simulink model "ThreePhaseInverter"  (R2019b)
settings: Solver=VariableStepAuto  StartTime=0.0  StopTime=1/50*20  RelTol=1e-9
undefined symbols (not defined in the file or in its folder): out
libraries: simulink x4, cstblocks x3
settings Model: Creator=reichyga  LastModifiedBy=reichyga
settings HardwareCC: ProdBitPerLong=64  ProdHWDeviceType=Intel->x86-64 (Linux 64)

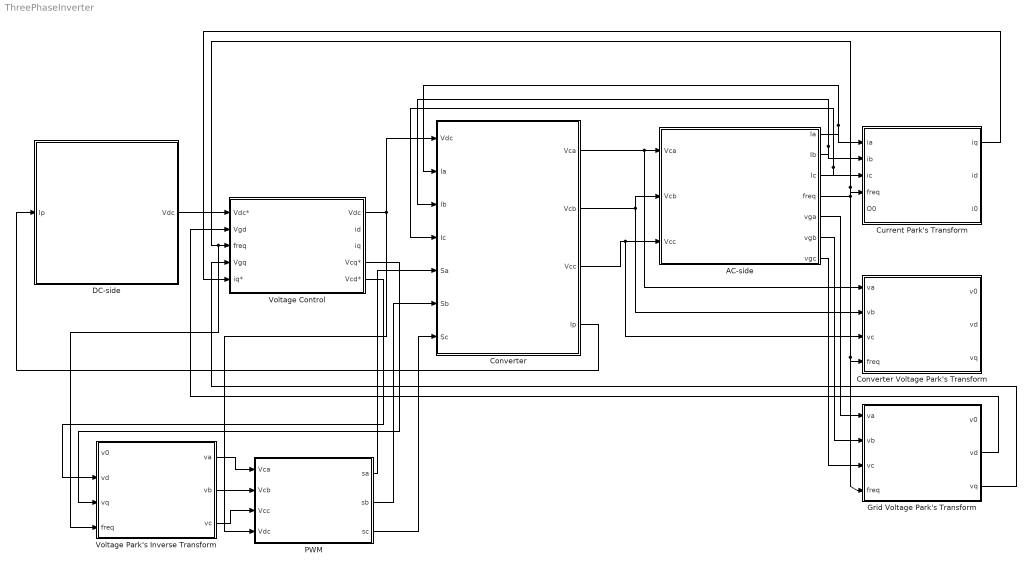
== system ThreePhaseInverter ==
  "AC-side " : Subsystem
  Converter : Subsystem
  Converter Voltage Park's Transform : Subsystem
  Current Park's Transform : Subsystem
  DC-side : Subsystem
  Grid Voltage Park's Transform : Subsystem
  PWM : Subsystem
  Voltage Control : Subsystem
  Voltage Park's Inverse Transform : Subsystem
  wires:
  "AC-side "/1(Ia) -> Converter/2(Ia), Current Park's Transform/1(ia)
  "AC-side "/3(Ic) -> Converter/4(Ic), Current Park's Transform/3(ic)
  Converter/1(Vca) -> Converter Voltage Park's Transform/1(va), "AC-side "/1("Vca ")
  Converter/2(Vcb) -> Converter Voltage Park's Transform/2(vb), "AC-side "/2(Vcb)
  Converter/3(Vcc) -> Converter Voltage Park's Transform/3(vc), "AC-side "/3(Vcc)
  Converter/4(Ip) -> DC-side/1(Ip)
  DC-side/1(Vdc) -> Voltage Control/1(Vdc*)
  "AC-side "/4(freq) -> Voltage Park's Inverse Transform/4("freq "), Voltage Control/3(freq), Current Park's Transform/4("freq "), Grid Voltage Park's Transform/4("freq "), Converter Voltage Park's Transform/4("freq ")
  "AC-side "/2(Ib) -> Converter/3(Ib), Current Park's Transform/2(ib)
  "AC-side "/5("vga ") -> Grid Voltage Park's Transform/1(va)
  "AC-side "/6(vgb) -> Grid Voltage Park's Transform/2(vb)
  "AC-side "/7("vgc ") -> Grid Voltage Park's Transform/3(vc)
  Grid Voltage Park's Transform/3(vq) -> Voltage Control/4(Vgq)
  Current Park's Transform/1("iq ") -> Voltage Control/5(iq*)
  Voltage Control/1(Vdc) -> PWM/4(Vdc), Converter/1(Vdc)
  Voltage Control/5(Vcd*) -> Voltage Park's Inverse Transform/2(vd)
  Voltage Control/4(Vcq*) -> Voltage Park's Inverse Transform/3(vq)
  Voltage Park's Inverse Transform/1("va ") -> PWM/1(Vca)
  Voltage Park's Inverse Transform/2(vb) -> PWM/2(Vcb)
  Voltage Park's Inverse Transform/3(vc) -> PWM/3(Vcc)
  PWM/1("sa ") -> Converter/5(Sa)
  PWM/2(sb) -> Converter/6(Sb)
  PWM/3(sc) -> Converter/7(Sc)
  Grid Voltage Park's Transform/2(vd) -> Voltage Control/2(Vgd)

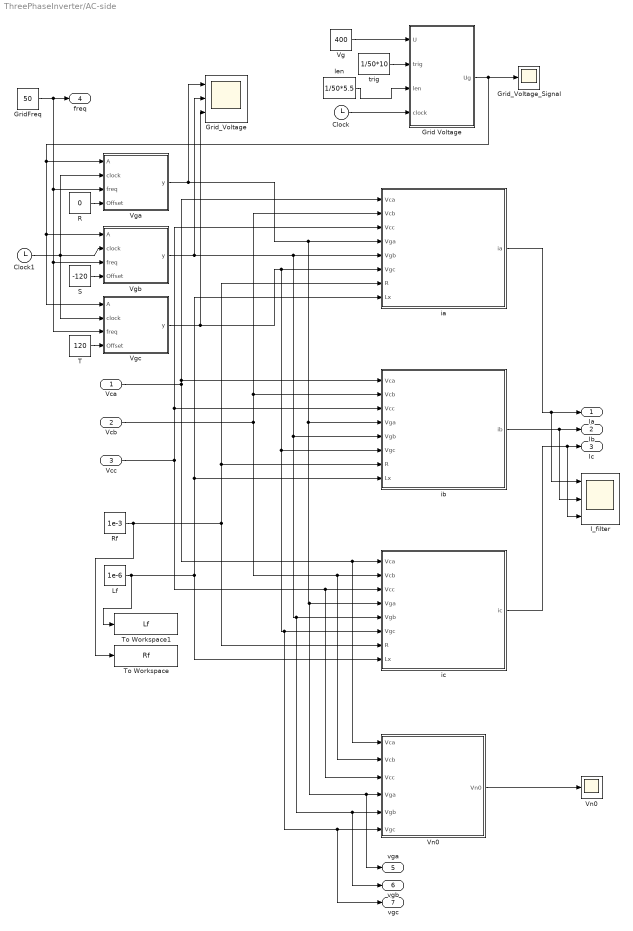
== system ThreePhaseInverter/AC-side  ==
  "Vca " : Inport
  Vcb : Inport  Port=2
  Vcc : Inport  Port=3
  Clock : Clock
  Clock1 : Clock
  Grid Voltage : MATLAB Function  TreatAsAtomicUnit=on
  "GridFreq " : Constant  Value=50
  Grid_Voltage : Scope  NumInputPorts=3
  "Grid_Voltage_Signal " : Scope
  I_filter : Scope  NumInputPorts=3
  "Lf " : Constant  Value=1e-6
  R : Constant  Value=0
  "Rf " : Constant  Value=1e-3
  S : Constant  Value=-120
  T : Constant  Value=120
  To Workspace : ToWorkspace  VariableName=Rf  SaveFormat=Timeseries  SampleTime=-1
  To Workspace1 : ToWorkspace  VariableName=Lf  SaveFormat=Timeseries  SampleTime=-1
  Vg : Constant  Value=400
  Vga : MATLAB Function  TreatAsAtomicUnit=on
  "Vgb " : MATLAB Function  TreatAsAtomicUnit=on
  Vgc : MATLAB Function  TreatAsAtomicUnit=on
  Vn0 : Subsystem
  "Vn0 " : Scope
  ia : Subsystem
  ib : Subsystem
  ic : Subsystem
  len : Constant  Value=1/50*5.5
  "trig " : Constant  Value=1/50*10
  Ia : Outport
  Ib : Outport  Port=2
  Ic : Outport  Port=3
  freq : Outport  Port=4
  "vga " : Outport  Port=5
  vgb : Outport  Port=6
  "vgc " : Outport  Port=7
  wires:
  Vn0/1("Vn0 ") -> "Vn0 "/1
  R/1 -> Vga/4(Offset)
  "Lf "/1 -> To Workspace1/1, ic/8(Lx), ib/8(Lx), ia/8(Lx)
  "Vca "/1 -> ib/1("Vca "), ia/1("Vca "), Vn0/1("Vca "), ic/1("Vca ")
  "Rf "/1 -> To Workspace/1, ib/7(R), ia/7(R), ic/7(R)
  Clock1/1 -> Vgc/2(clock), "Vgb "/2(clock), Vga/2(clock)
  Vcb/1 -> ib/2(Vcb), ia/2(Vcb), Vn0/2(Vcb), ic/2(Vcb)
  ic/1(ic) -> I_filter/3, Ic/1
  T/1 -> Vgc/4(Offset)
  ib/1(ib) -> I_filter/2, Ib/1
  Vg/1 -> Grid Voltage/1(U)
  Grid Voltage/1(Ug) -> Vgc/1(A), "Vgb "/1(A), Vga/1(A), "Grid_Voltage_Signal "/1
  Clock/1 -> Grid Voltage/4(clock)
  Vga/1(y) -> Grid_Voltage/1, "vga "/1, Vn0/4(Vga), ic/4(Vga), ib/4(Vga), ia/4(Vga)
  "Vgb "/1(y) -> Grid_Voltage/2, vgb/1, Vn0/5(Vgb), ic/5(Vgb), ib/5(Vgb), ia/5(Vgb)
  "trig "/1 -> Grid Voltage/2(trig)
  Vcc/1 -> Vn0/3(Vcc), ic/3(Vcc), ib/3(Vcc), ia/3(Vcc)
  "GridFreq "/1 -> Vga/3(freq), "Vgb "/3(freq), Vgc/3(freq), freq/1
  len/1 -> Grid Voltage/3(len)
  Vgc/1(y) -> Grid_Voltage/3, "vgc "/1, Vn0/6(Vgc), ic/6(Vgc), ib/6(Vgc), ia/6(Vgc)
  S/1 -> "Vgb "/4(Offset)
  ia/1(ia) -> I_filter/1, Ia/1

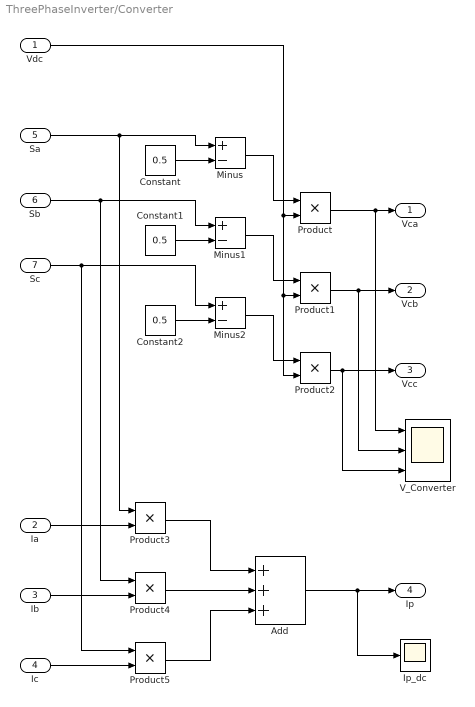
== system ThreePhaseInverter/Converter ==
  Vdc : Inport
  Ia : Inport  Port=2
  Ib : Inport  Port=3
  Ic : Inport  Port=4
  Sa : Inport  Port=5
  Sb : Inport  Port=6
  Sc : Inport  Port=7
  Add : Sum  Inputs=3
  Constant : Constant  Value=0.5
  Constant1 : Constant  Value=0.5
  Constant2 : Constant  Value=0.5
  Ip_dc : Scope
  Minus : Sum  Inputs=+-
  Minus1 : Sum  Inputs=+-
  Minus2 : Sum  Inputs=+-
  Product{,1..5} (6 alike) : Product
  V_Converter : Scope  NumInputPorts=3
  Vca : Outport
  Vcb : Outport  Port=2
  Vcc : Outport  Port=3
  Ip : Outport  Port=4
  wires:
  Constant/1 -> Minus/2
  Minus/1 -> Product/1
  Vdc/1 -> Product2/2, Product1/2, Product/2
  Product/1 -> V_Converter/1, Vca/1
  Minus1/1 -> Product1/1
  Constant1/1 -> Minus1/2
  Sb/1 -> Product4/1, Minus1/1
  Constant2/1 -> Minus2/2
  Minus2/1 -> Product2/1
  Sc/1 -> Product5/1, Minus2/1
  Product1/1 -> V_Converter/2, Vcb/1
  Product2/1 -> V_Converter/3, Vcc/1
  Sa/1 -> Product3/1, Minus/1
  Ia/1 -> Product3/2
  Ib/1 -> Product4/2
  Ic/1 -> Product5/2
  Product5/1 -> Add/3
  Product4/1 -> Add/2
  Product3/1 -> Add/1
  Add/1 -> Ip_dc/1, Ip/1

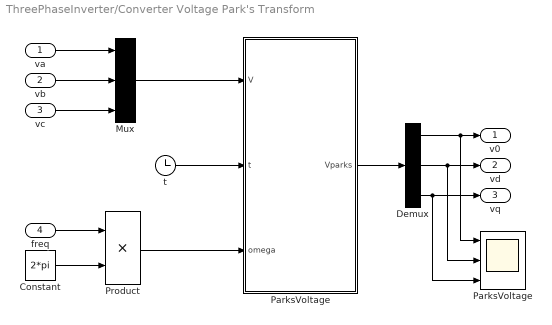
== system ThreePhaseInverter/Converter Voltage Park's Transform ==
  va : Inport
  vb : Inport  Port=2
  vc : Inport  Port=3
  "freq " : Inport  Port=4
  Constant : Constant  Value=2*pi
  Demux : Demux  Outputs=3
  Mux : Mux  Inputs=3
  ParksVoltage : MATLAB Function  TreatAsAtomicUnit=on
  "ParksVoltage " : Scope  NumInputPorts=3
  Product : Product
  t : Clock
  "v0 " : Outport
  vd : Outport  Port=2
  vq : Outport  Port=3
  wires:
  va/1 -> Mux/1
  vb/1 -> Mux/2
  vc/1 -> Mux/3
  Mux/1 -> ParksVoltage/1(V)
  "freq "/1 -> Product/1
  Product/1 -> ParksVoltage/3(omega)
  ParksVoltage/1(Vparks) -> Demux/1
  Demux/1 -> "ParksVoltage "/1, "v0 "/1
  Demux/2 -> "ParksVoltage "/2, vd/1
  Demux/3 -> vq/1, "ParksVoltage "/3
  Constant/1 -> Product/2
  t/1 -> ParksVoltage/2(t)

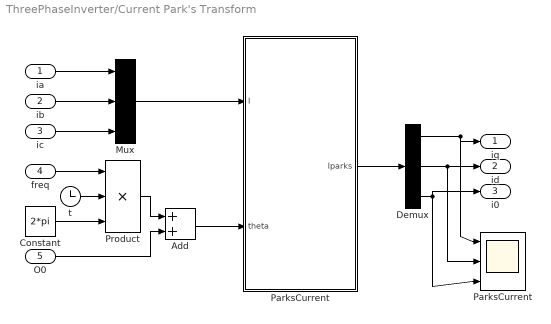
== system ThreePhaseInverter/Current Park's Transform ==
  ia : Inport
  ib : Inport  Port=2
  ic : Inport  Port=3
  "freq " : Inport  Port=4
  "O0 " : Inport  Port=5
  Add : Sum
  Constant : Constant  Value=2*pi
  Demux : Demux  Outputs=3
  Mux : Mux  Inputs=3
  ParksCurrent : MATLAB Function  TreatAsAtomicUnit=on
  "ParksCurrent " : Scope  NumInputPorts=3
  Product : Product  Inputs=3
  t : Clock
  "iq " : Outport
  id : Outport  Port=2
  i0 : Outport  Port=3
  wires:
  ia/1 -> Mux/1
  ib/1 -> Mux/2
  ic/1 -> Mux/3
  Mux/1 -> ParksCurrent/1(I)
  "freq "/1 -> Product/1
  t/1 -> Product/2
  "O0 "/1 -> Add/2
  Product/1 -> Add/1
  Add/1 -> ParksCurrent/2(theta)
  ParksCurrent/1(Iparks) -> Demux/1
  Demux/1 -> "ParksCurrent "/1, "iq "/1
  Demux/2 -> "ParksCurrent "/2, id/1
  Demux/3 -> i0/1, "ParksCurrent "/3
  Constant/1 -> Product/3

== system ThreePhaseInverter/DC-side ==
  Ip : Inport
  Constant1 : Constant  Value=inf
  Constant2 : Constant  Value=1e-6
  Constant3 : Constant  Value=1000
  Constant4 : Constant  Value=50
  To Workspace : ToWorkspace  VariableName=Idc  SaveFormat=Timeseries  SampleTime=-1
  To Workspace1 : ToWorkspace  VariableName=C  SaveFormat=Timeseries  SampleTime=-1
  V_DC-side : Scope
  "Vdc " : Subsystem
  Vdc : Outport
  wires:
  Ip/1 -> "Vdc "/4(Ip)
  Constant1/1 -> "Vdc "/3(Rp)
  Constant2/1 -> To Workspace1/1, "Vdc "/5(C)
  Constant3/1 -> "Vdc "/2(VdcIn)
  "Vdc "/1(Vdc) -> V_DC-side/1, Vdc/1
  Constant4/1 -> To Workspace/1, "Vdc "/1("Idc ")

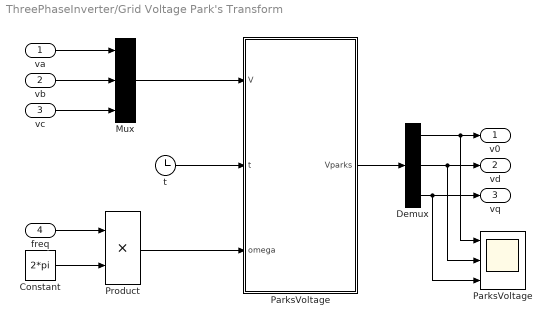
== system ThreePhaseInverter/Grid Voltage Park's Transform ==
  va : Inport
  vb : Inport  Port=2
  vc : Inport  Port=3
  "freq " : Inport  Port=4
  Constant : Constant  Value=2*pi
  Demux : Demux  Outputs=3
  Mux : Mux  Inputs=3
  ParksVoltage : MATLAB Function  TreatAsAtomicUnit=on
  "ParksVoltage " : Scope  NumInputPorts=3
  Product : Product
  t : Clock
  "v0 " : Outport
  vd : Outport  Port=2
  vq : Outport  Port=3
  wires:
  va/1 -> Mux/1
  vb/1 -> Mux/2
  vc/1 -> Mux/3
  Mux/1 -> ParksVoltage/1(V)
  "freq "/1 -> Product/1
  Product/1 -> ParksVoltage/3(omega)
  ParksVoltage/1(Vparks) -> Demux/1
  Demux/1 -> "ParksVoltage "/1, "v0 "/1
  Demux/2 -> "ParksVoltage "/2, vd/1
  Demux/3 -> vq/1, "ParksVoltage "/3
  Constant/1 -> Product/2
  t/1 -> ParksVoltage/2(t)

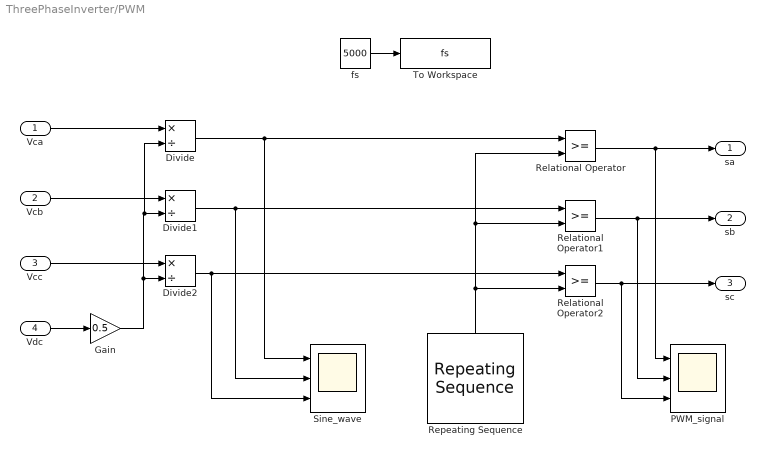
== system ThreePhaseInverter/PWM ==
  Vca : Inport
  Vcb : Inport  Port=2
  Vcc : Inport  Port=3
  Vdc : Inport  Port=4
  Divide : Product  Inputs=*/
  Divide1 : Product  Inputs=*/
  Divide2 : Product  Inputs=*/
  Gain : Gain  Gain=0.5
  PWM_signal : Scope  NumInputPorts=3
  Relational Operator : RelationalOperator  OutDataTypeStr=boolean  RndMeth=Simplest
  Relational Operator1 : RelationalOperator  OutDataTypeStr=boolean  RndMeth=Simplest
  Relational Operator2 : RelationalOperator  OutDataTypeStr=boolean  RndMeth=Simplest
  Repeating Sequence : simulink/Sources/Repeating Sequence  rep_seq_t=[0 (1/out.fs.Data)*0.25 (1/out.fs.Data)*0.75 (1/out.fs.Data)]  rep_seq_y=[0 -1 1 0]
  Sine_wave : Scope  NumInputPorts=3
  To Workspace : ToWorkspace  VariableName=fs  SaveFormat=Timeseries  SampleTime=-1
  fs : Constant  Value=5000
  "sa " : Outport
  sb : Outport  Port=2
  sc : Outport  Port=3
  wires:
  Vca/1 -> Divide/1
  Vcb/1 -> Divide1/1
  Vcc/1 -> Divide2/1
  Gain/1 -> Divide/2, Divide1/2, Divide2/2
  Divide/1 -> Sine_wave/1, Relational Operator/1
  Repeating Sequence/1 -> Relational Operator2/2, Relational Operator/2, Relational Operator1/2
  Divide1/1 -> Sine_wave/2, Relational Operator1/1
  Divide2/1 -> Sine_wave/3, Relational Operator2/1
  Vdc/1 -> Gain/1
  Relational Operator2/1 -> PWM_signal/3, sc/1
  Relational Operator1/1 -> PWM_signal/2, sb/1
  Relational Operator/1 -> PWM_signal/1, "sa "/1
  fs/1 -> To Workspace/1

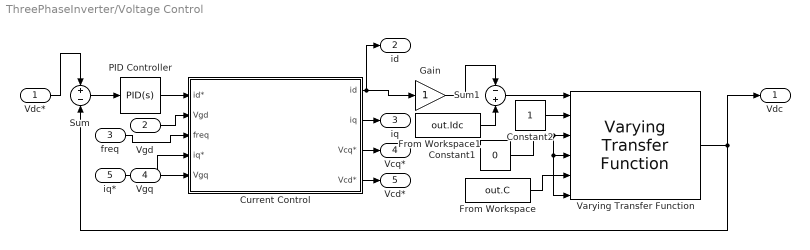
== system ThreePhaseInverter/Voltage Control ==
  Vdc* : Inport
  Vgd : Inport  Port=2
  freq : Inport  Port=3
  Vgq : Inport  Port=4
  iq* : Inport  Port=5
  Constant1 : Constant  Value=0
  Constant2 : Constant
  Current Control : Subsystem
  From Workspace : FromWorkspace  VariableName=out.C  SampleTime=0
  From Workspace1 : FromWorkspace  VariableName=out.Idc  SampleTime=0
  Gain : Gain
  PID Controller : simulink/Continuous/PID Controller  Controller=PID  Form=Parallel  TimeDomain=Continuous-time  SampleTime=-1  IntegratorMethod=Forward Euler  FilterMethod=Forward Euler  ControllerParametersSource=internal  P=1  I=1  D=0  UseFilter=on  N=100  TunerSelectOption=Transfer Function Based (PID Tuner App)  InitialConditionSource=internal  InitialConditionForIntegrator=0  InitialConditionForFilter=0  DifferentiatorICPrevScaledInput=0  ExternalReset=none  TrackingMode=off  Kt=1  LimitOutput=off  UpperSaturationLimit=inf  LowerSaturationLimit=-inf  LinearizeAsGain=on  AntiWindupMode=none  Kb=1  POutMin=[]  POutMax=[]  IOutMin=[]  IOutMax=[]  DOutMin=[]  DOutMax=[]  NOutMin=[]  NOutMax=[]  SumOutMin=[]  SumOutMax=[]  SaturationOutMin=[]  SaturationOutMax=[]  PParamMin=[]  PParamMax=[]  IParamMin=[]  IParamMax=[]  DParamMin=[]  DParamMax=[]  NParamMin=[]  NParamMax=[]  KbParamMin=[]  KbParamMax=[]  KtParamMin=[]  KtParamMax=[]  KbOutMin=[]  KbOutMax=[]  KtOutMin=[]  KtOutMax=[]  IntegratorOutMin=[]  IntegratorOutMax=[]  FilterOutMin=[]  FilterOutMax=[]  SumI1OutMin=[]  SumI1OutMax=[]  SumI2OutMin=[]  SumI2OutMax=[]  SumI3OutMin=[]  SumI3OutMax=[]  SumI4OutMin=[]  SumI4OutMax=[]  SumDOutMin=[]  SumDOutMax=[]  DifferentiatorOutMin=[]  DifferentiatorOutMax=[]  FilterDiffOutCoefMin=[]  FilterDiffOutCoefMax=[]  ReciprocalOutMin=[]  ReciprocalOutMax=[]  SumDenOutMin=[]  SumDenOutMax=[]  SumNumOutMin=[]  SumNumOutMax=[]  DivideOutMin=[]  DivideOutMax=[]  IntegratorContinuousStateAttributes=''  IntegratorStateMustResolveToSignalObject=off  IntegratorRTWStateStorageClass=Auto  FilterContinuousStateAttributes=''  FilterStateMustResolveToSignalObject=off  FilterRTWStateStorageClass=Auto  ParallelPVariant=InternalParameters  IdealPVariant=Disabled  IVariant=InternalParameters  DVariant=InternalParameters  IntegratorVariant=Continuous  SatVariant=Disabled  AWVariant=Passthrough  PCopyVariant=Disabled  TRVariant=Disabled  FdbkBlocksVariant=Forward  IdealPFdbkVariant=Disabled  SatFdbkVariant=Disabled  DerivativeFilterVariant=ContFilter  NVariant=InternalParameters  NCopyVariant=Disabled  FilterICVariant=InternalICsFilter  IntegratorICVariant=InternalICs  ExternalResetVariant=Disabled  TRSumVariant=Passthrough  SumFdbkVariant=Disabled  SumVariant=Sum_PID
  Sum : Sum  Inputs=+-
  Sum1 : Sum  Inputs=-+
  Varying Transfer Function : cstblocks/Linear Parameter Varying/Varying Transfer Function  N=2
      settings: SourceProductName=Control System Toolbox
  Vdc : Outport
  id : Outport  Port=2
  iq : Outport  Port=3
  Vcq* : Outport  Port=4
  Vcd* : Outport  Port=5
  wires:
  From Workspace/1 -> Varying Transfer Function/5
  Vgd/1 -> Current Control/2(Vgd)
  Constant1/1 -> Varying Transfer Function/6, Varying Transfer Function/4, Varying Transfer Function/3
  Sum/1 -> PID Controller/1
  Sum1/1 -> Varying Transfer Function/1
  Varying Transfer Function/1 -> Vdc/1, Sum/2
  Constant2/1 -> Varying Transfer Function/2
  Vdc*/1 -> Sum/1
  PID Controller/1 -> Current Control/1(id*)
  Current Control/1(id) -> id/1, Gain/1
  freq/1 -> Current Control/3("freq ")
  Vgq/1 -> Current Control/5(Vgq)
  Gain/1 -> Sum1/1
  From Workspace1/1 -> Sum1/2
  iq*/1 -> Current Control/4(iq*)
  Current Control/2(iq) -> iq/1
  Current Control/3(Vcq*) -> Vcq*/1
  Current Control/4(Vcd*) -> Vcd*/1

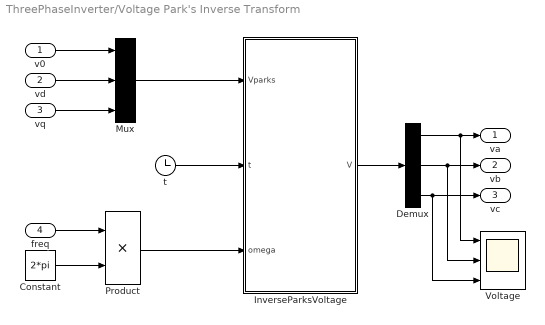
== system ThreePhaseInverter/Voltage Park's Inverse Transform ==
  v0 : Inport
  vd : Inport  Port=2
  vq : Inport  Port=3
  "freq " : Inport  Port=4
  Constant : Constant  Value=2*pi
  Demux : Demux  Outputs=3
  InverseParksVoltage : MATLAB Function  TreatAsAtomicUnit=on
  Mux : Mux  Inputs=3
  Product : Product
  "Voltage " : Scope  NumInputPorts=3
  t : Clock
  "va " : Outport
  vb : Outport  Port=2
  vc : Outport  Port=3
  wires:
  v0/1 -> Mux/1
  vd/1 -> Mux/2
  vq/1 -> Mux/3
  Mux/1 -> InverseParksVoltage/1(Vparks)
  "freq "/1 -> Product/1
  Product/1 -> InverseParksVoltage/3(omega)
  InverseParksVoltage/1(V) -> Demux/1
  Demux/1 -> "Voltage "/1, "va "/1
  Demux/2 -> "Voltage "/2, vb/1
  Demux/3 -> vc/1, "Voltage "/3
  Constant/1 -> Product/2
  t/1 -> InverseParksVoltage/2(t)

== system ThreePhaseInverter/AC-side /Vn0 ==
  "Vca " : Inport
  Vcb : Inport  Port=2
  Vcc : Inport  Port=3
  Vga : Inport  Port=4
  Vgb : Inport  Port=5
  Vgc : Inport  Port=6
  Add : Sum  Inputs=+++
  Add1 : Sum  Inputs=3
  Constant : Constant  Value=3
  Divide : Product  Inputs=*/
  Subtract : Sum  Inputs=+-
  "Vn0 " : Outport
  wires:
  "Vca "/1 -> Add1/1
  Vcb/1 -> Add1/2
  Vcc/1 -> Add1/3
  Vga/1 -> Add/1
  Vgb/1 -> Add/2
  Vgc/1 -> Add/3
  Add1/1 -> Subtract/1
  Add/1 -> Subtract/2
  Subtract/1 -> Divide/1
  Constant/1 -> Divide/2
  Divide/1 -> "Vn0 "/1

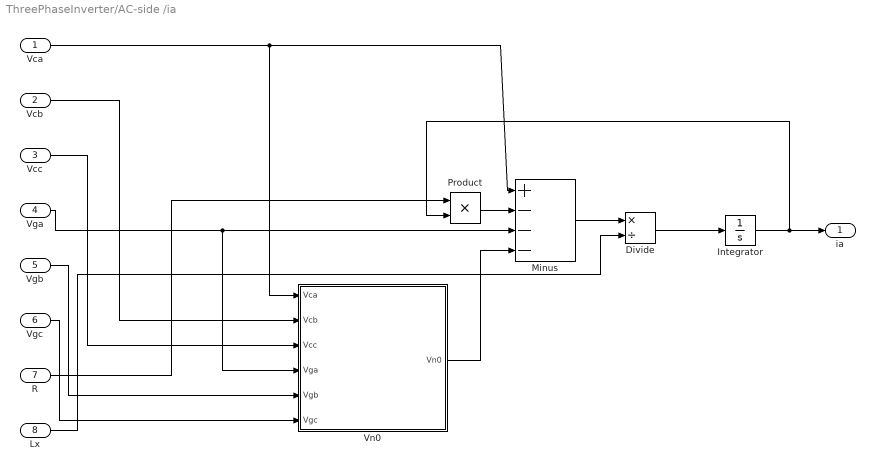
== system ThreePhaseInverter/AC-side /ia ==
  "Vca " : Inport
  Vcb : Inport  Port=2
  Vcc : Inport  Port=3
  Vga : Inport  Port=4
  Vgb : Inport  Port=5
  Vgc : Inport  Port=6
  R : Inport  Port=7
  Lx : Inport  Port=8
  Divide : Product  Inputs=*/
  Integrator : Integrator
  Minus : Sum  Inputs=+---
  Product : Product
  Vn0 : Subsystem
  ia : Outport
  wires:
  "Vca "/1 -> Vn0/1("Vca "), Minus/1
  Vga/1 -> Vn0/4(Vga), Minus/3
  Vcb/1 -> Vn0/2(Vcb)
  Vcc/1 -> Vn0/3(Vcc)
  Vgb/1 -> Vn0/5(Vgb)
  Vgc/1 -> Vn0/6(Vgc)
  Vn0/1("Vn0 ") -> Minus/4
  Minus/1 -> Divide/1
  Lx/1 -> Divide/2
  Divide/1 -> Integrator/1
  Integrator/1 -> Product/2, ia/1
  R/1 -> Product/1
  Product/1 -> Minus/2

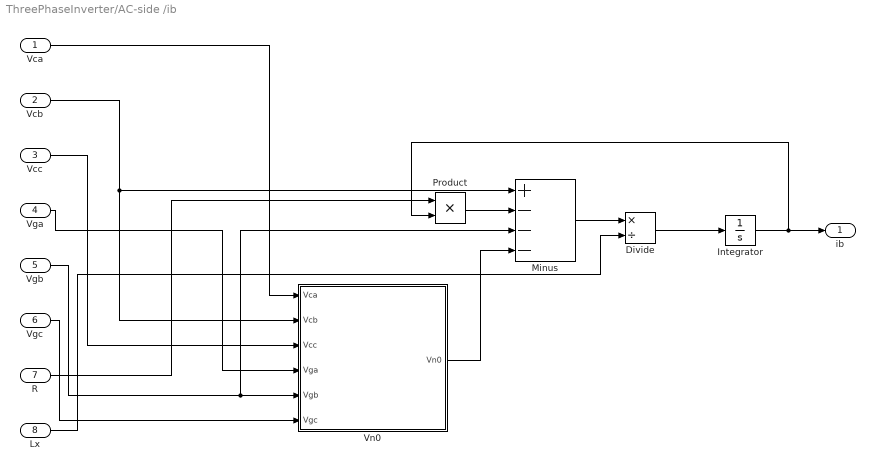
== system ThreePhaseInverter/AC-side /ib ==
  "Vca " : Inport
  Vcb : Inport  Port=2
  Vcc : Inport  Port=3
  Vga : Inport  Port=4
  Vgb : Inport  Port=5
  Vgc : Inport  Port=6
  R : Inport  Port=7
  Lx : Inport  Port=8
  Divide : Product  Inputs=*/
  Integrator : Integrator
  Minus : Sum  Inputs=+---
  Product : Product
  Vn0 : Subsystem
  ib : Outport
  wires:
  "Vca "/1 -> Vn0/1("Vca ")
  Vga/1 -> Vn0/4(Vga)
  Vcb/1 -> Minus/1, Vn0/2(Vcb)
  Vcc/1 -> Vn0/3(Vcc)
  Vgb/1 -> Minus/3, Vn0/5(Vgb)
  Vgc/1 -> Vn0/6(Vgc)
  Vn0/1("Vn0 ") -> Minus/4
  Minus/1 -> Divide/1
  Lx/1 -> Divide/2
  Divide/1 -> Integrator/1
  Integrator/1 -> Product/2, ib/1
  R/1 -> Product/1
  Product/1 -> Minus/2

== system ThreePhaseInverter/AC-side /ic ==
  "Vca " : Inport
  Vcb : Inport  Port=2
  Vcc : Inport  Port=3
  Vga : Inport  Port=4
  Vgb : Inport  Port=5
  Vgc : Inport  Port=6
  R : Inport  Port=7
  Lx : Inport  Port=8
  Divide : Product  Inputs=*/
  Integrator : Integrator
  Minus : Sum  Inputs=+---
  Product : Product
  Vn0 : Subsystem
  ic : Outport
  wires:
  "Vca "/1 -> Vn0/1("Vca ")
  Vga/1 -> Vn0/4(Vga)
  Vcb/1 -> Vn0/2(Vcb)
  Vcc/1 -> Minus/1, Vn0/3(Vcc)
  Vgb/1 -> Vn0/5(Vgb)
  Vgc/1 -> Minus/3, Vn0/6(Vgc)
  Vn0/1("Vn0 ") -> Minus/4
  Minus/1 -> Divide/1
  Lx/1 -> Divide/2
  Divide/1 -> Integrator/1
  Integrator/1 -> Product/2, ic/1
  R/1 -> Product/1
  Product/1 -> Minus/2

== system ThreePhaseInverter/DC-side/Vdc  ==
  "Idc " : Inport
  VdcIn : Inport  Port=2
  Rp : Inport  Port=3
  Ip : Inport  Port=4
  C : Inport  Port=5
  Divide : Product  Inputs=*/
  Divide1 : Product  Inputs=*/
  Integrator : Integrator  InitialCondition=1000
  Minus : Sum  Inputs=+--
  Vdc : Outport
  wires:
  Minus/1 -> Divide1/1
  Integrator/1 -> Vdc/1
  "Idc "/1 -> Minus/1
  Divide1/1 -> Integrator/1
  Divide/1 -> Minus/2
  Ip/1 -> Minus/3
  VdcIn/1 -> Divide/1
  Rp/1 -> Divide/2
  C/1 -> Divide1/2

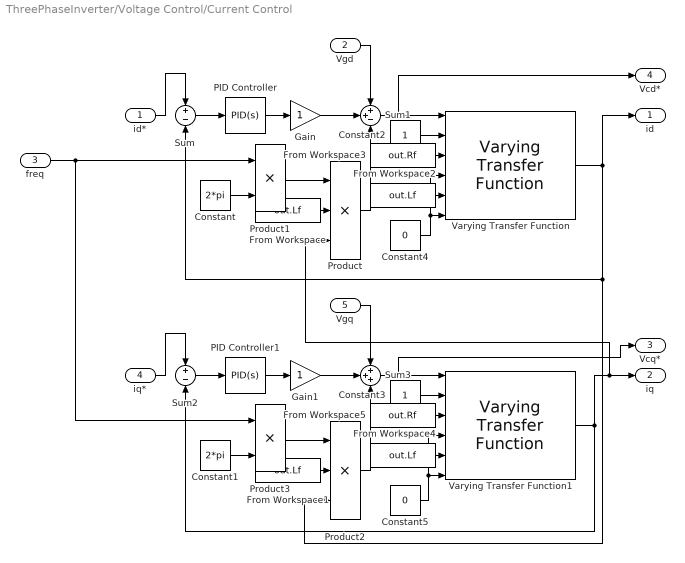
== system ThreePhaseInverter/Voltage Control/Current Control ==
  id* : Inport
  Vgd : Inport  Port=2
  "freq " : Inport  Port=3
  iq* : Inport  Port=4
  Vgq : Inport  Port=5
  Constant : Constant  Value=2*pi
  Constant1 : Constant  Value=2*pi
  Constant2 : Constant
  Constant3 : Constant
  Constant4 : Constant  Value=0
  Constant5 : Constant  Value=0
  From Workspace{,1..2,4} (4 alike) : FromWorkspace  VariableName=out.Lf  SampleTime=0
  From Workspace3 : FromWorkspace  VariableName=out.Rf  SampleTime=0
  From Workspace5 : FromWorkspace  VariableName=out.Rf  SampleTime=0
  Gain : Gain
  Gain1 : Gain
  PID Controller : simulink/Continuous/PID Controller  Controller=PID  Form=Parallel  TimeDomain=Continuous-time  SampleTime=-1  IntegratorMethod=Forward Euler  FilterMethod=Forward Euler  ControllerParametersSource=internal  P=1  I=1  D=0  UseFilter=on  N=100  TunerSelectOption=Transfer Function Based (PID Tuner App)  InitialConditionSource=internal  InitialConditionForIntegrator=0  InitialConditionForFilter=0  DifferentiatorICPrevScaledInput=0  ExternalReset=none  TrackingMode=off  Kt=1  LimitOutput=off  UpperSaturationLimit=inf  LowerSaturationLimit=-inf  LinearizeAsGain=on  AntiWindupMode=none  Kb=1  POutMin=[]  POutMax=[]  IOutMin=[]  IOutMax=[]  DOutMin=[]  DOutMax=[]  NOutMin=[]  NOutMax=[]  SumOutMin=[]  SumOutMax=[]  SaturationOutMin=[]  SaturationOutMax=[]  PParamMin=[]  PParamMax=[]  IParamMin=[]  IParamMax=[]  DParamMin=[]  DParamMax=[]  NParamMin=[]  NParamMax=[]  KbParamMin=[]  KbParamMax=[]  KtParamMin=[]  KtParamMax=[]  KbOutMin=[]  KbOutMax=[]  KtOutMin=[]  KtOutMax=[]  IntegratorOutMin=[]  IntegratorOutMax=[]  FilterOutMin=[]  FilterOutMax=[]  SumI1OutMin=[]  SumI1OutMax=[]  SumI2OutMin=[]  SumI2OutMax=[]  SumI3OutMin=[]  SumI3OutMax=[]  SumI4OutMin=[]  SumI4OutMax=[]  SumDOutMin=[]  SumDOutMax=[]  DifferentiatorOutMin=[]  DifferentiatorOutMax=[]  FilterDiffOutCoefMin=[]  FilterDiffOutCoefMax=[]  ReciprocalOutMin=[]  ReciprocalOutMax=[]  SumDenOutMin=[]  SumDenOutMax=[]  SumNumOutMin=[]  SumNumOutMax=[]  DivideOutMin=[]  DivideOutMax=[]  IntegratorContinuousStateAttributes=''  IntegratorStateMustResolveToSignalObject=off  IntegratorRTWStateStorageClass=Auto  FilterContinuousStateAttributes=''  FilterStateMustResolveToSignalObject=off  FilterRTWStateStorageClass=Auto  ParallelPVariant=InternalParameters  IdealPVariant=Disabled  IVariant=InternalParameters  DVariant=InternalParameters  IntegratorVariant=Continuous  SatVariant=Disabled  AWVariant=Passthrough  PCopyVariant=Disabled  TRVariant=Disabled  FdbkBlocksVariant=Forward  IdealPFdbkVariant=Disabled  SatFdbkVariant=Disabled  DerivativeFilterVariant=ContFilter  NVariant=InternalParameters  NCopyVariant=Disabled  FilterICVariant=InternalICsFilter  IntegratorICVariant=InternalICs  ExternalResetVariant=Disabled  TRSumVariant=Passthrough  SumFdbkVariant=Disabled  SumVariant=Sum_PID
  PID Controller1 : simulink/Continuous/PID Controller  Controller=PID  Form=Parallel  TimeDomain=Continuous-time  SampleTime=-1  IntegratorMethod=Forward Euler  FilterMethod=Forward Euler  ControllerParametersSource=internal  P=1  I=1  D=0  UseFilter=on  N=100  TunerSelectOption=Transfer Function Based (PID Tuner App)  InitialConditionSource=internal  InitialConditionForIntegrator=0  InitialConditionForFilter=0  DifferentiatorICPrevScaledInput=0  ExternalReset=none  TrackingMode=off  Kt=1  LimitOutput=off  UpperSaturationLimit=inf  LowerSaturationLimit=-inf  LinearizeAsGain=on  AntiWindupMode=none  Kb=1  POutMin=[]  POutMax=[]  IOutMin=[]  IOutMax=[]  DOutMin=[]  DOutMax=[]  NOutMin=[]  NOutMax=[]  SumOutMin=[]  SumOutMax=[]  SaturationOutMin=[]  SaturationOutMax=[]  PParamMin=[]  PParamMax=[]  IParamMin=[]  IParamMax=[]  DParamMin=[]  DParamMax=[]  NParamMin=[]  NParamMax=[]  KbParamMin=[]  KbParamMax=[]  KtParamMin=[]  KtParamMax=[]  KbOutMin=[]  KbOutMax=[]  KtOutMin=[]  KtOutMax=[]  IntegratorOutMin=[]  IntegratorOutMax=[]  FilterOutMin=[]  FilterOutMax=[]  SumI1OutMin=[]  SumI1OutMax=[]  SumI2OutMin=[]  SumI2OutMax=[]  SumI3OutMin=[]  SumI3OutMax=[]  SumI4OutMin=[]  SumI4OutMax=[]  SumDOutMin=[]  SumDOutMax=[]  DifferentiatorOutMin=[]  DifferentiatorOutMax=[]  FilterDiffOutCoefMin=[]  FilterDiffOutCoefMax=[]  ReciprocalOutMin=[]  ReciprocalOutMax=[]  SumDenOutMin=[]  SumDenOutMax=[]  SumNumOutMin=[]  SumNumOutMax=[]  DivideOutMin=[]  DivideOutMax=[]  IntegratorContinuousStateAttributes=''  IntegratorStateMustResolveToSignalObject=off  IntegratorRTWStateStorageClass=Auto  FilterContinuousStateAttributes=''  FilterStateMustResolveToSignalObject=off  FilterRTWStateStorageClass=Auto  ParallelPVariant=InternalParameters  IdealPVariant=Disabled  IVariant=InternalParameters  DVariant=InternalParameters  IntegratorVariant=Continuous  SatVariant=Disabled  AWVariant=Passthrough  PCopyVariant=Disabled  TRVariant=Disabled  FdbkBlocksVariant=Forward  IdealPFdbkVariant=Disabled  SatFdbkVariant=Disabled  DerivativeFilterVariant=ContFilter  NVariant=InternalParameters  NCopyVariant=Disabled  FilterICVariant=InternalICsFilter  IntegratorICVariant=InternalICs  ExternalResetVariant=Disabled  TRSumVariant=Passthrough  SumFdbkVariant=Disabled  SumVariant=Sum_PID
  Product : Product  Inputs=3
  Product1 : Product
  Product2 : Product  Inputs=3
  Product3 : Product
  Sum : Sum  Inputs=+-
  Sum1 : Sum  Inputs=++-
  Sum2 : Sum  Inputs=+-
  Sum3 : Sum  Inputs=+++
  Varying Transfer Function : cstblocks/Linear Parameter Varying/Varying Transfer Function  N=2
      settings: SourceProductName=Control System Toolbox
  Varying Transfer Function1 : cstblocks/Linear Parameter Varying/Varying Transfer Function  N=2
      settings: SourceProductName=Control System Toolbox
  id : Outport
  iq : Outport  Port=2
  Vcq* : Outport  Port=3
  Vcd* : Outport  Port=4
  wires:
  id*/1 -> Sum/1
  Sum/1 -> PID Controller/1
  PID Controller/1 -> Gain/1
  Gain/1 -> Sum1/2
  Vgd/1 -> Sum1/1
  Product/1 -> Sum1/3
  Product1/1 -> Product/1
  Constant/1 -> Product1/2
  From Workspace/1 -> Product/2
  Sum1/1 -> Vcd*/1, Varying Transfer Function/1
  Varying Transfer Function/1 -> id/1, Sum/2, Product2/3
  Gain1/1 -> Sum3/2
  iq*/1 -> Sum2/1
  Product3/1 -> Product2/1
  From Workspace1/1 -> Product2/2
  Product2/1 -> Sum3/3
  Varying Transfer Function1/1 -> Product/3, iq/1, Sum2/2
  Vgq/1 -> Sum3/1
  Sum2/1 -> PID Controller1/1
  Constant1/1 -> Product3/2
  "freq "/1 -> Product3/1, Product1/1
  PID Controller1/1 -> Gain1/1
  Constant2/1 -> Varying Transfer Function/2
  From Workspace2/1 -> Varying Transfer Function/5
  From Workspace3/1 -> Varying Transfer Function/3
  Constant3/1 -> Varying Transfer Function1/2
  From Workspace5/1 -> Varying Transfer Function1/3
  From Workspace4/1 -> Varying Transfer Function1/5
  Sum3/1 -> Vcq*/1, Varying Transfer Function1/1
  Constant4/1 -> Varying Transfer Function/4, Varying Transfer Function/6
  Constant5/1 -> Varying Transfer Function1/6, Varying Transfer Function1/4

== system ThreePhaseInverter/AC-side /ia/Vn0 ==
  "Vca " : Inport
  Vcb : Inport  Port=2
  Vcc : Inport  Port=3
  Vga : Inport  Port=4
  Vgb : Inport  Port=5
  Vgc : Inport  Port=6
  Add : Sum  Inputs=+++
  Add1 : Sum  Inputs=3
  Constant : Constant  Value=3
  Divide : Product  Inputs=*/
  Subtract : Sum  Inputs=+-
  "Vn0 " : Outport
  wires:
  "Vca "/1 -> Add1/1
  Vcb/1 -> Add1/2
  Vcc/1 -> Add1/3
  Vga/1 -> Add/1
  Vgb/1 -> Add/2
  Vgc/1 -> Add/3
  Add1/1 -> Subtract/1
  Add/1 -> Subtract/2
  Subtract/1 -> Divide/1
  Constant/1 -> Divide/2
  Divide/1 -> "Vn0 "/1

== system ThreePhaseInverter/AC-side /ib/Vn0 ==
  "Vca " : Inport
  Vcb : Inport  Port=2
  Vcc : Inport  Port=3
  Vga : Inport  Port=4
  Vgb : Inport  Port=5
  Vgc : Inport  Port=6
  Add : Sum  Inputs=+++
  Add1 : Sum  Inputs=3
  Constant : Constant  Value=3
  Divide : Product  Inputs=*/
  Subtract : Sum  Inputs=+-
  "Vn0 " : Outport
  wires:
  "Vca "/1 -> Add1/1
  Vcb/1 -> Add1/2
  Vcc/1 -> Add1/3
  Vga/1 -> Add/1
  Vgb/1 -> Add/2
  Vgc/1 -> Add/3
  Add1/1 -> Subtract/1
  Add/1 -> Subtract/2
  Subtract/1 -> Divide/1
  Constant/1 -> Divide/2
  Divide/1 -> "Vn0 "/1

== system ThreePhaseInverter/AC-side /ic/Vn0 ==
  "Vca " : Inport
  Vcb : Inport  Port=2
  Vcc : Inport  Port=3
  Vga : Inport  Port=4
  Vgb : Inport  Port=5
  Vgc : Inport  Port=6
  Add : Sum  Inputs=+++
  Add1 : Sum  Inputs=3
  Constant : Constant  Value=3
  Divide : Product  Inputs=*/
  Subtract : Sum  Inputs=+-
  "Vn0 " : Outport
  wires:
  "Vca "/1 -> Add1/1
  Vcb/1 -> Add1/2
  Vcc/1 -> Add1/3
  Vga/1 -> Add/1
  Vgb/1 -> Add/2
  Vgc/1 -> Add/3
  Add1/1 -> Subtract/1
  Add/1 -> Subtract/2
  Subtract/1 -> Divide/1
  Constant/1 -> Divide/2
  Divide/1 -> "Vn0 "/1

== matlab function ThreePhaseInverter/AC-side /Vga ==
  data: A input; y output; clock input; freq input; Offset input
function y = SineWave(A,clock,freq,Offset) %Amplitude, simClock, frequency in Hz, Offset in degree
    
y=A*sin(2*pi*freq*clock+Offset/180*pi);

== matlab function ThreePhaseInverter/AC-side /Grid Voltage ==
  data: U input; Ug output; trig input; len input; clock input
function Ug = tempFault(U,trig,len,clock)
    if or(clock<trig,clock>(trig+len))
        Ug=U;
    else
        Ug=U/2;
    end

== matlab function ThreePhaseInverter/AC-side /Vgb  ==
  data: A input; y output; clock input; freq input; Offset input
function y = SineWave(A,clock,freq,Offset) %Amplitude, simClock, frequency in Hz, Offset in degree
    
y=A*sin(2*pi*freq*clock+Offset/180*pi);

== matlab function ThreePhaseInverter/AC-side /Vgc ==
  data: A input; y output; clock input; freq input; Offset input
function y = SineWave(A,clock,freq,Offset) %Amplitude, simClock, frequency in Hz, Offset in degree
    
y=A*sin(2*pi*freq*clock+Offset/180*pi);

== matlab function ThreePhaseInverter/Current Park's Transform/ParksCurrent ==
  data: I input; Iparks output; theta input
function Iparks=parks_current(I,theta)
    Iparks=2/3*[cos(theta),cos(theta-120/180*pi),cos(theta+120/180*pi);
        sin(theta),sin(theta-120/180*pi),sin(theta+120/180*pi);
        .5,.5,.5]*I;

== matlab function ThreePhaseInverter/Converter Voltage Park's Transform/ParksVoltage ==
  data: V input; Vparks output; t input; omega input
function Vparks=parks_voltage(V,t,omega)
    Vparks=sqrt(2/3)*[1/sqrt(2),1/sqrt(2),1/sqrt(2);
        cos(omega*t),cos(omega*t-(2*pi)/(3)),cos(omega*t+(2*pi)/(3));
        -sin(omega*t),-sin(omega*t-(2*pi)/(3)),-sin(omega*t+(2*pi)/(3))]*V;

== matlab function ThreePhaseInverter/Grid Voltage Park's Transform/ParksVoltage ==
  data: V input; Vparks output; t input; omega input
function Vparks=parks_voltage(V,t,omega)
    Vparks=sqrt(2/3)*[1/sqrt(2),1/sqrt(2),1/sqrt(2);
        cos(omega*t),cos(omega*t-(2*pi)/(3)),cos(omega*t+(2*pi)/(3));
        -sin(omega*t),-sin(omega*t-(2*pi)/(3)),-sin(omega*t+(2*pi)/(3))]*V;

== matlab function ThreePhaseInverter/Voltage Park's Inverse Transform/InverseParksVoltage ==
  data: Vparks input; V output; t input; omega input
function V=inverse_parks_voltage(Vparks,t,omega)
    V=sqrt(2/3)*[1/sqrt(2),1/sqrt(2),1/sqrt(2);
        cos(omega*t),cos(omega*t-(2*pi)/(3)),cos(omega*t+(2*pi)/(3));
        -sin(omega*t),-sin(omega*t-(2*pi)/(3)),-sin(omega*t+(2*pi)/(3))]\Vparks;
